simulink model "Efficiency_Map_SR_Validation_Sim"  (R2019a)
settings: Solver=VariableStepAuto  StartTime=0.0  StopTime=10.0  RelTol=1e-3
undefined symbols (not defined in the file or in its folder): ap00, ap01, ap02, ap03, ap10, ap11, ap12, ap20, ap21, ap30, motor_speed, motor_torque
settings Model: Creator=Robert Wygant  LastModifiedBy=hangking
settings DataIOCC: ReturnWorkspaceOutputs=off
settings DebuggingCC: ArithmeticOperatorsInVariantConditions=warning
settings SFSimCC: SimUseLocalCustomCode=off
settings RTWCC: RTWUseLocalCustomCode=off

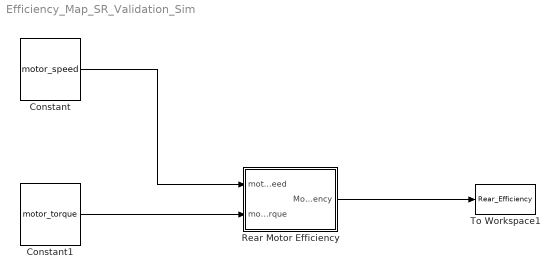
== system Efficiency_Map_SR_Validation_Sim ==
  Constant : Constant  Value=motor_speed  VectorParams1D=off
  Constant1 : Constant  Value=motor_torque
  Rear Motor Efficiency : Subsystem
      mask Display:
      | color('green')
      | disp("Motor Efficiency")
  To Workspace1 : ToWorkspace  VariableName=Rear_Efficiency  SampleTime=-1
      settings: MaxDataPoints=1  Save2DSignal=2-D array (concatenate along first dimension)
  wires:
  Constant/1 -> Rear Motor Efficiency/1(motor_speed)
  Constant1/1 -> Rear Motor Efficiency/2(motor_torque)
  Rear Motor Efficiency/1(Motor_efficiency) -> To Workspace1/1

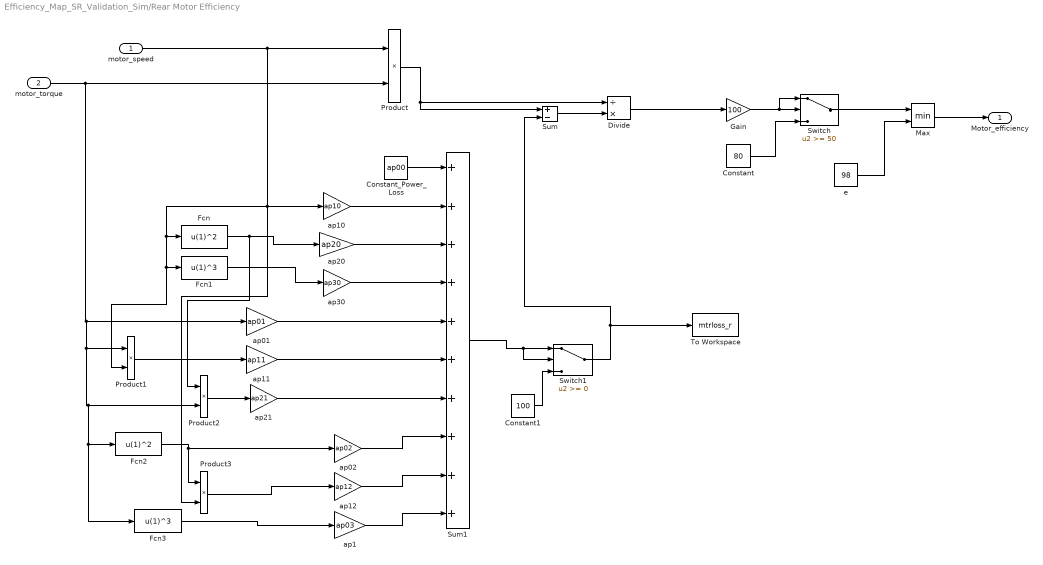
== system Efficiency_Map_SR_Validation_Sim/Rear Motor Efficiency ==
  motor_speed : Inport
  motor_torque : Inport  Port=2
  Constant : Constant  Value=80
  Constant1 : Constant  Value=100
  Constant_Power_Loss : Constant  Value=ap00
  Divide : Product  Inputs=/*
  Fcn : Fcn  Expr=u(1)^2
  Fcn1 : Fcn  Expr=u(1)^3
  Fcn2 : Fcn  Expr=u(1)^2
  Fcn3 : Fcn  Expr=u(1)^3
  Gain : Gain  Gain=100
  Max : MinMax  Inputs=2
  Product{,1..3} (4 alike) : Product
  Sum : Sum  Inputs=+-
  Sum1 : Sum  Inputs=++++++++++
  Switch : Switch  Threshold=50
  Switch1 : Switch
  To Workspace : ToWorkspace  VariableName=mtrloss_r  SampleTime=-1
      settings: MaxDataPoints=1  Save2DSignal=2-D array (concatenate along first dimension)
  ap01 : Gain  Gain=ap01
  ap02 : Gain  Gain=ap02
  ap1 : Gain  Gain=ap03
  ap10 : Gain  Gain=ap10
  ap11 : Gain  Gain=ap11
  ap12 : Gain  Gain=ap12
  ap20 : Gain  Gain=ap20
  ap21 : Gain  Gain=ap21
  ap30 : Gain  Gain=ap30
  e : Constant  Value=98
  Motor_efficiency : Outport
  wires:
  e/1 -> Max/2
  Fcn3/1 -> ap1/1
  ap1/1 -> Sum1/10
  ap12/1 -> Sum1/9
  Product3/1 -> ap12/1
  motor_torque/1 -> Product/2, Product1/1, Product2/2, Fcn2/1, Fcn3/1, ap01/1
  ap01/1 -> Sum1/5
  ap11/1 -> Sum1/6
  ap21/1 -> Sum1/7
  ap02/1 -> Sum1/8
  Fcn2/1 -> ap02/1, Product3/1
  Product2/1 -> ap21/1
  Product1/1 -> ap11/1
  ap30/1 -> Sum1/4
  Fcn1/1 -> ap30/1
  Fcn/1 -> ap20/1, Product2/1
  ap20/1 -> Sum1/3
  ap10/1 -> Sum1/2
  Constant_Power_Loss/1 -> Sum1/1
  motor_speed/1 -> Product/1, Product3/2, Fcn/1, Fcn1/1, Product1/2, ap10/1
  Product/1 -> Divide/1, Sum/1
  Constant/1 -> Switch/3
  Gain/1 -> Switch/1, Switch/2
  Divide/1 -> Gain/1
  Switch1/1 -> Sum/2, To Workspace/1
  Sum1/1 -> Switch1/2, Switch1/1
  Constant1/1 -> Switch1/3
  Sum/1 -> Divide/2
  Switch/1 -> Max/1
  Max/1 -> Motor_efficiency/1
